simulink model "dc_motor_pi"  (R2023a)
settings: Solver=VariableStepAuto  StartTime=0.0  StopTime=30  FixedStep=0.01  RelTol=1e-3
libraries: fuzblock x4, SignalEditorBlockLib x3, slpidlib x1
settings Model: Creator=eleft  LastModifiedBy=eleft

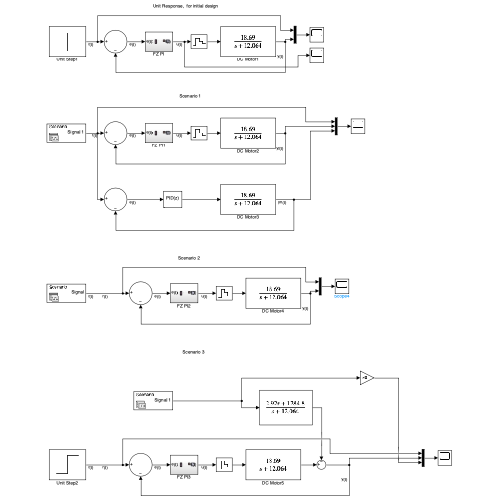
[thumbnail: Simulink's stored preview of the top-level diagram]
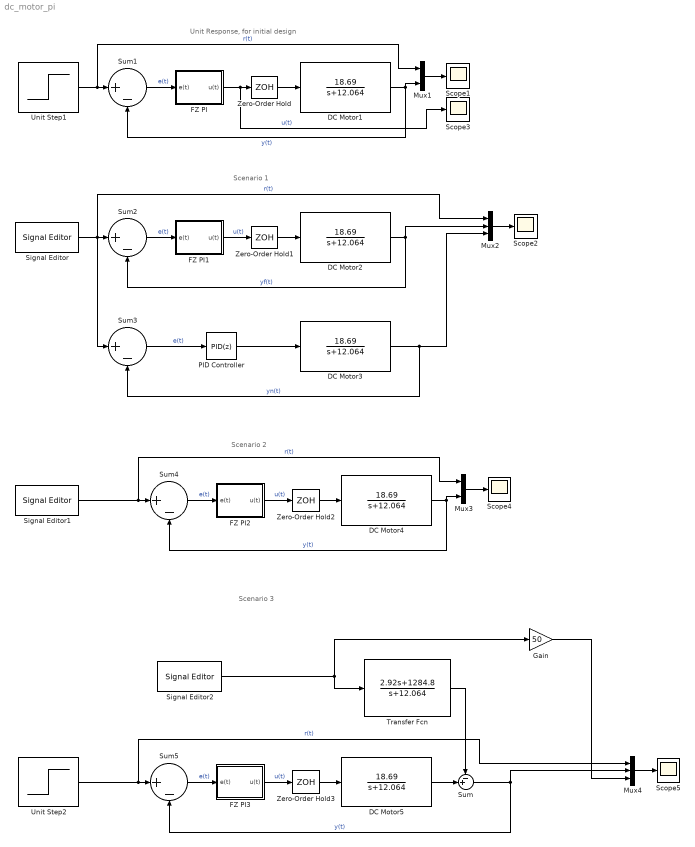
== system dc_motor_pi ==
  note: Scenario 1
  note: Unit Response, for initial design
  note: Scenario 2
  note: Scenario 3
  DC Motor{1..5} (5 alike) : TransferFcn  Numerator=[18.69]  Denominator=[1 12.064]
  FZ PI : Subsystem
  FZ PI1 : Subsystem
  FZ PI2 : Subsystem
  FZ PI3 : Subsystem
  Gain : Gain  Gain=50
  Mux1 : Mux  Inputs=2
  Mux2 : Mux  Inputs=3
  Mux3 : Mux  Inputs=2
  Mux4 : Mux  Inputs=3
  PID Controller : slpidlib/PID Controller  Controller=PID  Form=Parallel  TimeDomain=Discrete-time  UseExternalTs=off  SampleTime=0.01  IntegratorMethod=Forward Euler  FilterMethod=Forward Euler  ControllerParametersSource=internal  P=0.31011  I=8.1187  UseKiTs=off  D=0  N=100  UseFilter=on  TunerSelectOption=Transfer Function Based (PID Tuner App)  InitialConditionSource=internal  InitialConditionForIntegrator=0  InitialConditionForFilter=0  DifferentiatorICPrevScaledInput=0  ExternalReset=none  TrackingMode=off  Kt=1  LimitOutput=off  SatLimitsSource=internal  UpperSaturationLimit=inf  LowerSaturationLimit=-inf  LinearizeAsGain=on  AntiWindupMode=none  Kb=1  LimitIntegrator=off  UpperIntegratorSaturationLimit=inf  LowerIntegratorSaturationLimit=-inf  POutMin=[]  POutMax=[]  IOutMin=[]  IOutMax=[]  DOutMin=[]  DOutMax=[]  NOutMin=[]  NOutMax=[]  SumOutMin=[]  SumOutMax=[]  SaturationOutMin=[]  SaturationOutMax=[]  PParamMin=[]  PParamMax=[]  IParamMin=[]  IParamMax=[]  DParamMin=[]  DParamMax=[]  NParamMin=[]  NParamMax=[]  KbParamMin=[]  KbParamMax=[]  KtParamMin=[]  KtParamMax=[]  KbOutMin=[]  KbOutMax=[]  KtOutMin=[]  KtOutMax=[]  IntegratorOutMin=[]  IntegratorOutMax=[]  FilterOutMin=[]  FilterOutMax=[]  SumI1OutMin=[]  SumI1OutMax=[]  SumI2OutMin=[]  SumI2OutMax=[]  SumI3OutMin=[]  SumI3OutMax=[]  SumI4OutMin=[]  SumI4OutMax=[]  SumDOutMin=[]  SumDOutMax=[]  DifferentiatorOutMin=[]  DifferentiatorOutMax=[]  FilterDiffOutCoefMin=[]  FilterDiffOutCoefMax=[]  ReciprocalOutMin=[]  ReciprocalOutMax=[]  SumDenOutMin=[]  SumDenOutMax=[]  SumNumOutMin=[]  SumNumOutMax=[]  DivideOutMin=[]  DivideOutMax=[]  UdiffTsProdOutMin=[]  UdiffTsProdOutMax=[]  NTsProdOutMin=[]  NTsProdOutMax=[]  UintegralTsProdOutMin=[]  UintegralTsProdOutMax=[]  UngainTsProdOutMin=[]  UngainTsProdOutMax=[]  ClampingZeroOutDataTypeStr=Inherit: Inherit via back propagation  ClampingZeroOutMin=[]  ClampingZeroOutMax=[]  FilterDenConstantOutDataTypeStr=Inherit: Inherit via back propagation  FilterDenConstantOutMin=[]  FilterDenConstantOutMax=[]  PCopyOutDataTypeStr=Inherit: Inherit via back propagation  PCopyOutMin=[]  PCopyOutMax=[]  NCopyOutDataTypeStr=Inherit: Inherit via back propagation  NCopyOutMin=[]  NCopyOutMax=[]  IntegratorContinuousStateAttributes=''  IntegratorStateMustResolveToSignalObject=off  IntegratorRTWStateStorageClass=Auto  FilterContinuousStateAttributes=''  FilterStateMustResolveToSignalObject=off  FilterRTWStateStorageClass=Auto  ParallelPVariant=InternalParameters  IdealPVariant=Disabled  IVariant=InternalParameters  DVariant=InternalParameters  IntegratorVariant=Discrete  SatVariant=Disabled  AWVariant=Passthrough  PCopyVariant=Disabled  TRVariant=Disabled  FdbkBlocksVariant=Forward  IdealPFdbkVariant=Disabled  SatFdbkVariant=Disabled  DerivativeFilterVariant=ForwardEulerFilter  NVariant=InternalParameters  NCopyVariant=Disabled  FilterICVariant=InternalICsFilter  IntegratorICVariant=InternalICs  ExternalResetVariant=Disabled  TRSumVariant=Passthrough  SumFdbkVariant=Disabled  SumVariant=Sum_PID  TsampFilterVariant=InternalTs  TsampNgainVariant=Passthrough  TsampIntegralVariant=Disabled_SignalSpec  ExternalSaturationOutDataTypeStr=Inherit: Same as second input
  Scope{1..5} (5 alike) : Scope
  Signal Editor : SignalEditorBlockLib/Signal Editor  FileName=scenario1signal.mat  ActiveScenario=Scenario  ActiveSignal=Signal 1  IsBus=off  OutputBusObjectStr=Bus: BusObject  SampleTime=0.01  Interpolate=off  ZeroCross=off  OutputAfterFinalValue=Setting to zero  Unit=inherit  PreserveSignalName=on  ApplySigPropsToAllScenarios=on
  Signal Editor1 : SignalEditorBlockLib/Signal Editor  FileName=scenario2signal.mat  ActiveScenario=Scenario  ActiveSignal=Signal  IsBus=off  OutputBusObjectStr=Bus: BusObject  SampleTime=0.01  ZeroCross=off  OutputAfterFinalValue=Setting to zero  Unit=inherit  PreserveSignalName=on  ApplySigPropsToAllScenarios=on
  Signal Editor2 : SignalEditorBlockLib/Signal Editor  FileName=scenario3disturbance.mat  ActiveScenario=Scenario  ActiveSignal=Signal 1  IsBus=off  OutputBusObjectStr=Bus: BusObject  SampleTime=0.01  Interpolate=off  ZeroCross=off  OutputAfterFinalValue=Setting to zero  Unit=inherit  PreserveSignalName=on  ApplySigPropsToAllScenarios=on
  Sum : Sum  Inputs=-+|
  Sum{1..5} (5 alike) : Sum  Inputs=|+-
  Transfer Fcn : TransferFcn  Numerator=[2.92 1284.8]  Denominator=[1 12.064]
  Unit Step1 : Step  Time=0  After=150  SampleTime=0.01
  Unit Step2 : Step  Time=0  After=150  SampleTime=0.01
  Zero-Order Hold{,1..3} (4 alike) : ZeroOrderHold  SampleTime=0.01
  wires:
  DC Motor1/1 -> Mux1/2, Sum1/2  "y(t)"
  FZ PI/1(u(t)) -> Scope3/1, Zero-Order Hold/1  "u(t)"
  Mux1/1 -> Scope1/1
  Sum1/1 -> FZ PI/1(e(t))  "e(t)"
  Unit Step1/1 -> Mux1/1, Sum1/1  "r(t)"
  Zero-Order Hold/1 -> DC Motor1/1
  Sum2/1 -> FZ PI1/1(e(t))  "e(t)"
  DC Motor2/1 -> Mux2/2, Sum2/2  "yf(t)"
  FZ PI1/1(u(t)) -> Zero-Order Hold1/1  "u(t)"
  Mux2/1 -> Scope2/1
  Signal Editor/1 -> Mux2/1, Sum2/1, Sum3/1  "r(t)"
  Zero-Order Hold1/1 -> DC Motor2/1
  Sum3/1 -> PID Controller/1  "e(t)"
  PID Controller/1 -> DC Motor3/1
  DC Motor3/1 -> Sum3/2, Mux2/3  "yn(t)"
  Sum4/1 -> FZ PI2/1(e(t))  "e(t)"
  Zero-Order Hold2/1 -> DC Motor4/1
  DC Motor4/1 -> Mux3/2, Sum4/2  "y(t)"
  Mux3/1 -> Scope4/1
  FZ PI2/1(u(t)) -> Zero-Order Hold2/1  "u(t)"
  Signal Editor1/1 -> Mux3/1, Sum4/1  "r(t)"
  Unit Step2/1 -> Mux4/1, Sum5/1  "r(t)"
  Sum5/1 -> FZ PI3/1(e(t))  "e(t)"
  FZ PI3/1(u(t)) -> Zero-Order Hold3/1  "u(t)"
  DC Motor5/1 -> Sum/2
  Zero-Order Hold3/1 -> DC Motor5/1
  Mux4/1 -> Scope5/1
  Sum/1 -> Sum5/2, Mux4/2  "y(t)"
  Signal Editor2/1 -> Gain/1, Transfer Fcn/1
  Gain/1 -> Mux4/3
  Transfer Fcn/1 -> Sum/1

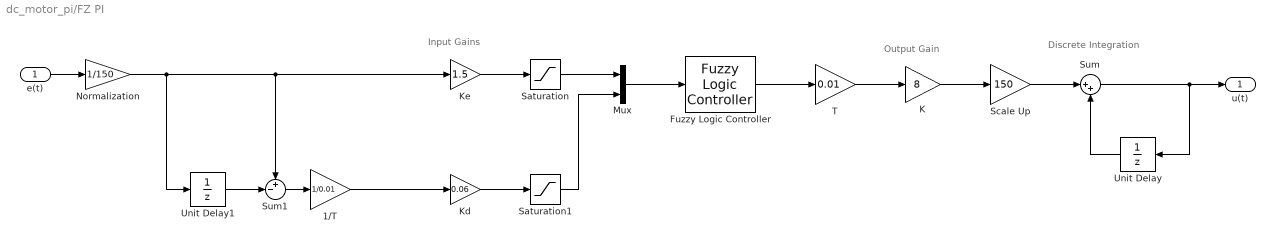
== system dc_motor_pi/FZ PI ==
  note: Input Gains
  note: Output Gain
  note: Discrete Integration
  e(t) : Inport
  1/T : Gain  Gain=1/0.01
  Fuzzy Logic Controller : fuzblock/Fuzzy Logic  Controller  FIS='fzcarcontrol.fis'  OutputSampleNumber=101  DataType=double  FuzzifiedInputs=off  RuleFiringStrengths=off  RuleOutputs=off  AggregatedOutputs=off  SimulateUsing=Interpreted execution  OutOfRangeInputValueMessage=warning  NoRuleFiredMessage=warning  EmptyOutputFuzzySetMessage=warning
  K : Gain  Gain=8
  Kd : Gain  Gain=0.06
  Ke : Gain  Gain=1.5
  Mux : Mux  Inputs=2
  Normalization : Gain  Gain=1/150
  Saturation : Saturate  UpperLimit=1  LowerLimit=-1
  Saturation1 : Saturate  UpperLimit=1  LowerLimit=-1
  Scale Up : Gain  Gain=150
  Sum : Sum  Inputs=|++
  Sum1 : Sum  Inputs=+-|
  T : Gain  Gain=0.01
  Unit Delay : UnitDelay  SampleTime=0.01  HasFrameUpgradeWarning=on
  Unit Delay1 : UnitDelay  SampleTime=0.01  HasFrameUpgradeWarning=on
  u(t) : Outport
  wires:
  Scale Up/1 -> Sum/1
  Unit Delay/1 -> Sum/2
  Sum/1 -> u(t)/1, Unit Delay/1
  K/1 -> Scale Up/1
  T/1 -> K/1
  Mux/1 -> Fuzzy Logic Controller/1
  Saturation/1 -> Mux/1
  Saturation1/1 -> Mux/2
  Ke/1 -> Saturation/1
  Unit Delay1/1 -> Sum1/2
  Kd/1 -> Saturation1/1
  Sum1/1 -> 1/T/1
  e(t)/1 -> Normalization/1
  1/T/1 -> Kd/1
  Normalization/1 -> Ke/1, Sum1/1, Unit Delay1/1
  Fuzzy Logic Controller/1 -> T/1

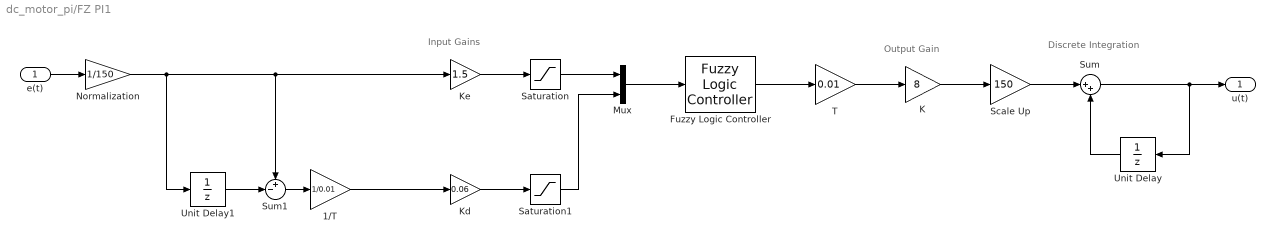
== system dc_motor_pi/FZ PI1 ==
  note: Input Gains
  note: Output Gain
  note: Discrete Integration
  e(t) : Inport
  1/T : Gain  Gain=1/0.01
  Fuzzy Logic Controller : fuzblock/Fuzzy Logic  Controller  FIS='fzcarcontrol.fis'  OutputSampleNumber=101  DataType=double  FuzzifiedInputs=off  RuleFiringStrengths=off  RuleOutputs=off  AggregatedOutputs=off  SimulateUsing=Interpreted execution  OutOfRangeInputValueMessage=warning  NoRuleFiredMessage=warning  EmptyOutputFuzzySetMessage=warning
  K : Gain  Gain=8
  Kd : Gain  Gain=0.06
  Ke : Gain  Gain=1.5
  Mux : Mux  Inputs=2
  Normalization : Gain  Gain=1/150
  Saturation : Saturate  UpperLimit=1  LowerLimit=-1
  Saturation1 : Saturate  UpperLimit=1  LowerLimit=-1
  Scale Up : Gain  Gain=150
  Sum : Sum  Inputs=|++
  Sum1 : Sum  Inputs=+-|
  T : Gain  Gain=0.01
  Unit Delay : UnitDelay  SampleTime=0.01  HasFrameUpgradeWarning=on
  Unit Delay1 : UnitDelay  SampleTime=0.01  HasFrameUpgradeWarning=on
  u(t) : Outport
  wires:
  Scale Up/1 -> Sum/1
  Unit Delay/1 -> Sum/2
  Sum/1 -> u(t)/1, Unit Delay/1
  K/1 -> Scale Up/1
  T/1 -> K/1
  Mux/1 -> Fuzzy Logic Controller/1
  Saturation/1 -> Mux/1
  Saturation1/1 -> Mux/2
  Ke/1 -> Saturation/1
  Unit Delay1/1 -> Sum1/2
  Kd/1 -> Saturation1/1
  Sum1/1 -> 1/T/1
  e(t)/1 -> Normalization/1
  1/T/1 -> Kd/1
  Normalization/1 -> Ke/1, Sum1/1, Unit Delay1/1
  Fuzzy Logic Controller/1 -> T/1

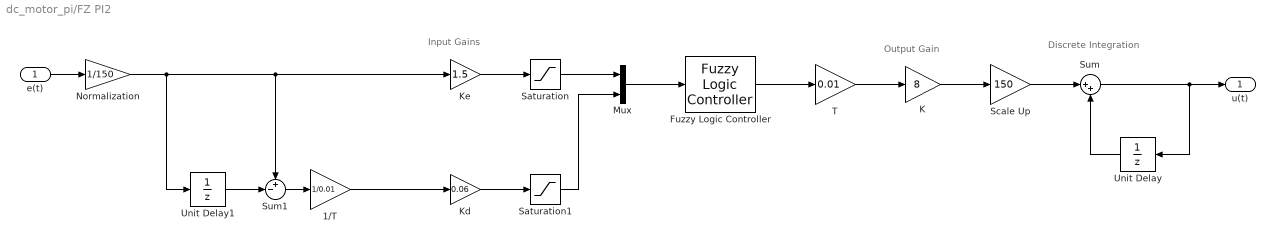
== system dc_motor_pi/FZ PI2 ==
  note: Input Gains
  note: Output Gain
  note: Discrete Integration
  e(t) : Inport
  1/T : Gain  Gain=1/0.01
  Fuzzy Logic Controller : fuzblock/Fuzzy Logic  Controller  FIS='fzcarcontrol.fis'  OutputSampleNumber=101  DataType=double  FuzzifiedInputs=off  RuleFiringStrengths=off  RuleOutputs=off  AggregatedOutputs=off  SimulateUsing=Interpreted execution  OutOfRangeInputValueMessage=warning  NoRuleFiredMessage=warning  EmptyOutputFuzzySetMessage=warning
  K : Gain  Gain=8
  Kd : Gain  Gain=0.06
  Ke : Gain  Gain=1.5
  Mux : Mux  Inputs=2
  Normalization : Gain  Gain=1/150
  Saturation : Saturate  UpperLimit=1  LowerLimit=-1
  Saturation1 : Saturate  UpperLimit=1  LowerLimit=-1
  Scale Up : Gain  Gain=150
  Sum : Sum  Inputs=|++
  Sum1 : Sum  Inputs=+-|
  T : Gain  Gain=0.01
  Unit Delay : UnitDelay  SampleTime=0.01  HasFrameUpgradeWarning=on
  Unit Delay1 : UnitDelay  SampleTime=0.01  HasFrameUpgradeWarning=on
  u(t) : Outport
  wires:
  Scale Up/1 -> Sum/1
  Unit Delay/1 -> Sum/2
  Sum/1 -> u(t)/1, Unit Delay/1
  K/1 -> Scale Up/1
  T/1 -> K/1
  Mux/1 -> Fuzzy Logic Controller/1
  Saturation/1 -> Mux/1
  Saturation1/1 -> Mux/2
  Ke/1 -> Saturation/1
  Unit Delay1/1 -> Sum1/2
  Kd/1 -> Saturation1/1
  Sum1/1 -> 1/T/1
  e(t)/1 -> Normalization/1
  1/T/1 -> Kd/1
  Normalization/1 -> Ke/1, Sum1/1, Unit Delay1/1
  Fuzzy Logic Controller/1 -> T/1

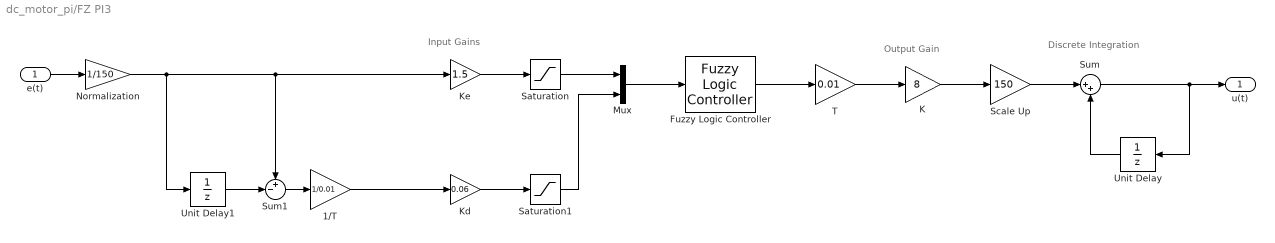
== system dc_motor_pi/FZ PI3 ==
  note: Input Gains
  note: Output Gain
  note: Discrete Integration
  e(t) : Inport
  1/T : Gain  Gain=1/0.01
  Fuzzy Logic Controller : fuzblock/Fuzzy Logic  Controller  FIS='fzcarcontrol.fis'  OutputSampleNumber=101  DataType=double  FuzzifiedInputs=off  RuleFiringStrengths=off  RuleOutputs=off  AggregatedOutputs=off  SimulateUsing=Interpreted execution  OutOfRangeInputValueMessage=warning  NoRuleFiredMessage=warning  EmptyOutputFuzzySetMessage=warning
  K : Gain  Gain=8
  Kd : Gain  Gain=0.06
  Ke : Gain  Gain=1.5
  Mux : Mux  Inputs=2
  Normalization : Gain  Gain=1/150
  Saturation : Saturate  UpperLimit=1  LowerLimit=-1
  Saturation1 : Saturate  UpperLimit=1  LowerLimit=-1
  Scale Up : Gain  Gain=150
  Sum : Sum  Inputs=|++
  Sum1 : Sum  Inputs=+-|
  T : Gain  Gain=0.01
  Unit Delay : UnitDelay  SampleTime=0.01  HasFrameUpgradeWarning=on
  Unit Delay1 : UnitDelay  SampleTime=0.01  HasFrameUpgradeWarning=on
  u(t) : Outport
  wires:
  Scale Up/1 -> Sum/1
  Unit Delay/1 -> Sum/2
  Sum/1 -> u(t)/1, Unit Delay/1
  K/1 -> Scale Up/1
  T/1 -> K/1
  Mux/1 -> Fuzzy Logic Controller/1
  Saturation/1 -> Mux/1
  Saturation1/1 -> Mux/2
  Ke/1 -> Saturation/1
  Unit Delay1/1 -> Sum1/2
  Kd/1 -> Saturation1/1
  Sum1/1 -> 1/T/1
  e(t)/1 -> Normalization/1
  1/T/1 -> Kd/1
  Normalization/1 -> Ke/1, Sum1/1, Unit Delay1/1
  Fuzzy Logic Controller/1 -> T/1
